simulink model "MotDynoReferenceApplication"  (R2023a)
settings: Solver=VariableStepAuto  StartTime=0.0  StopTime=36  RelTol=1e-3
libraries: simulink x2, autolibinverter x2, autolibmotorctrlr x2, autolibpowerinfoutils x1, autolibpmsminterior x1, autolibfluxpmsm x1, autolibmappedmotor x1
(part 7 of 7)

== system MotDynoReferenceApplication/Motor System/Motor Controller/Interior PM Controller SS Trq ==
  MotTrqCmd : Inport
  MotSpd : Inport  Port=2
  MotPlnt : Inport  Port=3
  BusVolt : Inport  Port=4
  Bus Creator : BusCreator  Inputs=3
  Bus Selector1 : BusSelector  OutputSignals=IaStator,IbStator,MtrPos
  Interior PM Controller SS Trq : autolibmotorctrlr/Interior PM Controller  VariantControl=Dynamic Motor Model  control_type=Torque Control  Rs=0.0096  Ld=0.00024276  Lq=0.00036413  lambda_pm=0.1331  PolePairs=4  Mechanical=Mechanical  MotorConstraint=Maximum Torque  T_max=347  I_max=44  bp=10  T_mtpa=[0 36.3756979805622 72.9371938225984 109.862728657458 147.316831782547 185.446415278493 224.379215188327 264.224116249109 305.072683110981 347.001277652692]  id_mtpa=[0 -1.88218850549476 -7.45328588922809 -16.5012550115386 -28.7146572298234 -43.7288523957444 -61.1678393829391 -80.6742871506256 -101.926636240741 -124.645868377109]  iq_mtpa=[0 45.4712908563859 90.7147850811458 135.529837727677 179.761962805355 223.30989814842 266.122168845454 308.187483121614 349.523304044935 390.165429631501]  idq_limits=[-124.648282637394 390.164658341277 409.592059228468]  EV_current=200  Tst=5e-5  Kp_d=0.30506  Kp_q=0.45758  Ki=12.0637  EV_motion=EV_motion  EV_sf=EV_sf  ba=ba  Ksa=Ksa  Kisa=Kisa  Ksf=Ksf  Jcomp=Jcomp  Fv=Fv  Fs=Fs  param_loss=Single efficiency measurement  eff=98  w_loss_bp=[0 200 400 600 800 1000]  T_loss_bp=[0 25 50 75 100]  losses_table=[100 100 100 100 100;100 150 200 250 300;100 200 300 400 500;100 250 400 550 700;100 300 500 700 900;100 350 600 850 1100]  w_eff_bp=[200 400 600 800 1000]  T_eff_bp=[25 50 75 100]  efficiency_table=[96.2 98.1 98.7 99;98.1 99 99.4 99.5;98.7 99.4 99.6 99.7;99 99.5 99.7 99.8;99.2 99.6 99.7 99.8]  x_w_bp=[-1000 -800 -600 -400 -200 200 400 600 800 1000]  x_T_bp=[-100 -75 -50 -25 25 50 75 100]  x_losses_mat=[200.400801603196 225.67703109328 200.803212851408 201.612903225806 199.999999999997 200 225 200;160.320641282556 180.541624874624 201.005025125625 202.020202020203 200 200 180 160;180.541624874624 180.722891566267 181.086519114686 197.568389057748 194.999999999999 179.999999999997 180 180;201.005025125625 181.086519114686 202.020202020203 193.67991845056 190 200 179.999999999997 200;202.020202020203 197.568389057748 193.67991845056 197.505197505197 190 190 194.999999999999 200;200 194.999999999999 190 190 197.505197505197 193.67991845056 197.568389057748 202.020202020203;200 179.999999999997 200 190 193.67991845056 202.020202020203 181.086519114686 201.005025125625;180 180 179.999999999997 194.999999999999 197.568389057748 181.086519114686 180.722891566267 180.541624874624;160 180 200 200 202.020202020203 201.005025125625 180.541624874624 160.320641282556;200 225 200 199.999999999997 201.612903225806 200.803212851408 225.67703109328 200.400801603196]  Tsm=5e-4
  MotCtrlr : Outport  VectorParamsAs1DForOutWhenUnconnected=off
  wires:
  Interior PM Controller SS Trq/3 -> Bus Creator/3  "PhaseVolt"
  MotTrqCmd/1 -> Interior PM Controller SS Trq/1  "MotTrqCmd"
  MotSpd/1 -> Interior PM Controller SS Trq/5
  MotPlnt/1 -> Bus Selector1/1
  Bus Selector1/1 -> Interior PM Controller SS Trq/3  "<IaStator>"
  Bus Selector1/2 -> Interior PM Controller SS Trq/4  "<IbStator>"
  Bus Selector1/3 -> Interior PM Controller SS Trq/6  "<MtrPos>"
  Interior PM Controller SS Trq/2 -> Bus Creator/2  "BusCurr"
  Interior PM Controller SS Trq/1 -> Bus Creator/1  "Info"
  BusVolt/1 -> Interior PM Controller SS Trq/2
  Bus Creator/1 -> MotCtrlr/1

== system MotDynoReferenceApplication/Motor System/Motor Controller/Mapped Motor Controller ==
  MotTrqCmd : Inport
  MotSpd : Inport  Port=2
  MotPlnt : Inport  Port=3
  BusVolt : Inport  Port=4
  Bus Creator : BusCreator  Inputs=3
  Mapped Motor Controller : Subsystem
  MotCtrlr : Outport  VectorParamsAs1DForOutWhenUnconnected=off
  wires:
  MotTrqCmd/1 -> Mapped Motor Controller/1(MotTrqCmd)  "MotTrqCmd"
  BusVolt/1 -> Mapped Motor Controller/2(BusVolt)
  MotPlnt/1 -> Mapped Motor Controller/3(MotPlnt)
  MotSpd/1 -> Mapped Motor Controller/4(SpdFdbk)
  Mapped Motor Controller/1(Info) -> Bus Creator/1
  Mapped Motor Controller/2(BusCurr) -> Bus Creator/2
  Mapped Motor Controller/3(PhaseVolt) -> Bus Creator/3
  Bus Creator/1 -> MotCtrlr/1

== system MotDynoReferenceApplication/Motor System/Motor & Inverter Plant/Mapped Motor Model/Info_Compatibility ==
  MtrSpd : Inport
  Info : Inport  Port=2
  Idc : Inport  Port=3
  MtrTrq : Inport  Port=4
  Bus Creator : BusCreator  Inputs=7
  Bus Selector1 : BusSelector  OutputSignals=MechPwr,PwrLoss,PwrInfo
  Dummy Values : Constant  Value=0
  Info_ : Outport
  wires:
  MtrSpd/1 -> Bus Creator/3  "MtrSpd"
  Bus Selector1/1 -> Bus Creator/5  "<MechPwr>"
  MtrTrq/1 -> Bus Creator/4  "MtrTrq"
  Info/1 -> Bus Selector1/1
  Dummy Values/1 -> Bus Creator/1  "IdSync"
  Bus Selector1/3 -> Bus Creator/7  "<PwrInfo>"
  Bus Selector1/2 -> Bus Creator/6  "<PwrLoss>"
  Idc/1 -> Bus Creator/2  "IqSync"
  Bus Creator/1 -> Info_/1

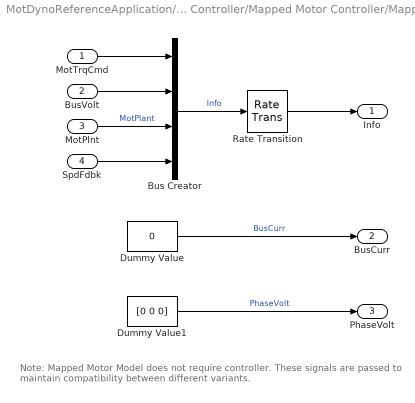
== system MotDynoReferenceApplication/Motor System/Motor Controller/Mapped Motor Controller/Mapped Motor Controller ==
  note: Note:
      | Mapped Motor Model does not require controller.
      | These signals are passed to maintain compatibility between different variants.
  MotTrqCmd : Inport
  BusVolt : Inport  Port=2
  MotPlnt : Inport  Port=3
  SpdFdbk : Inport  Port=4
  Bus Creator : BusCreator  Inputs=4
  Dummy Value : Constant  Value=0  SampleTime=-1
  Dummy Value1 : Constant  Value=[0 0 0]  SampleTime=-1
  Rate Transition : RateTransition  InitialCondition=-1
  Info : Outport
  BusCurr : Outport  Port=2
  PhaseVolt : Outport  Port=3
  wires:
  SpdFdbk/1 -> Bus Creator/4
  BusVolt/1 -> Bus Creator/2
  MotTrqCmd/1 -> Bus Creator/1
  Bus Creator/1 -> Rate Transition/1  "Info"
  Dummy Value/1 -> BusCurr/1  "BusCurr"
  Dummy Value1/1 -> PhaseVolt/1  "PhaseVolt"
  MotPlnt/1 -> Bus Creator/3  "MotPlant"
  Rate Transition/1 -> Info/1
